simulink model "HighwayLaneFollowingController"  (R2024a)
settings: configuration reference "csMultiInstance" (kept outside this file)
Description:
  | The integrated SW component of highway lane following controller
settings Model: DataDictionary=DD_HLF.sldd  EnableAccessToBaseWorkspace=off  Creator=The MathWorks, Inc.  LastModifiedBy=The MathWorks, Inc.
settings ConfigSetRef: SourceName=csMultiInstance

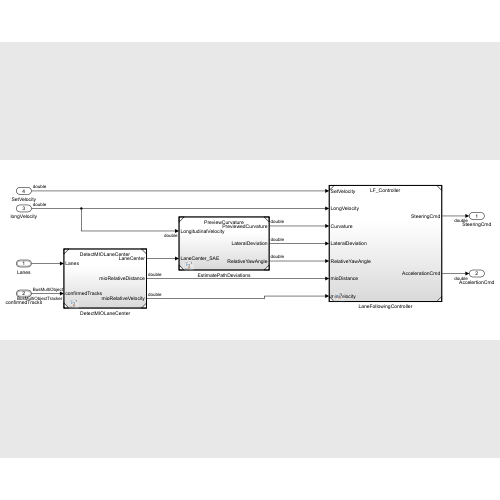
[thumbnail: Simulink's stored preview of the top-level diagram]
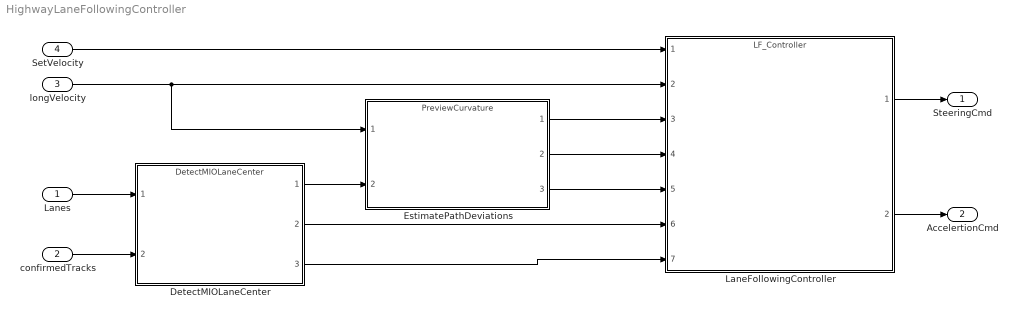
== system HighwayLaneFollowingController ==
  Lanes : Inport  OutDataTypeStr=Bus: LaneSensor
  confirmedTracks : Inport  Port=2  OutDataTypeStr=Bus: BusMultiObjectTracker  BusOutputAsStruct=on
  longVelocity : Inport  Port=3  OutDataTypeStr=Velocity_DType
  SetVelocity : Inport  Port=4  OutDataTypeStr=Velocity_DType
  DetectMIOLaneCenter : ModelReference  ModelNameDialog=DetectMIOLaneCenter  SimulationMode=Normal  ModelReferenceVersion=8.0
  EstimatePathDeviations : ModelReference  ModelNameDialog=PreviewCurvature  SimulationMode=Normal  ModelReferenceVersion=8.0
  LaneFollowingController : ModelReference  ModelNameDialog=LF_Controller  SimulationMode=Normal  ModelReferenceVersion=8.0
  SteeringCmd : Outport  OutDataTypeStr=Steering_DType
  AccelertionCmd : Outport  Port=2  OutDataTypeStr=Acceleration_DType
  wires:
  LaneFollowingController/1 -> SteeringCmd/1
  LaneFollowingController/2 -> AccelertionCmd/1
  Lanes/1 -> DetectMIOLaneCenter/1
  confirmedTracks/1 -> DetectMIOLaneCenter/2
  longVelocity/1 -> EstimatePathDeviations/1, LaneFollowingController/2
  SetVelocity/1 -> LaneFollowingController/1
  EstimatePathDeviations/3 -> LaneFollowingController/5
  EstimatePathDeviations/2 -> LaneFollowingController/4
  EstimatePathDeviations/1 -> LaneFollowingController/3
  DetectMIOLaneCenter/1 -> EstimatePathDeviations/2
  DetectMIOLaneCenter/3 -> LaneFollowingController/7
  DetectMIOLaneCenter/2 -> LaneFollowingController/6
